simulink model "Neurofeedback_Fuzzy_full_fNIRS_pressure"  (R2022a)
settings: Solver=VariableStepAuto  StartTime=0.0  StopTime=200  RelTol=1e-6
libraries: fuzblock x1, simulink x1
settings Model: Creator=mariodelossantos  LastModifiedBy=mariodelossantos

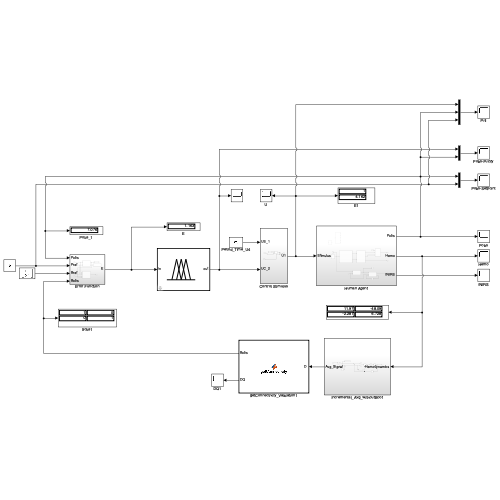
[thumbnail: Simulink's stored preview of the top-level diagram]
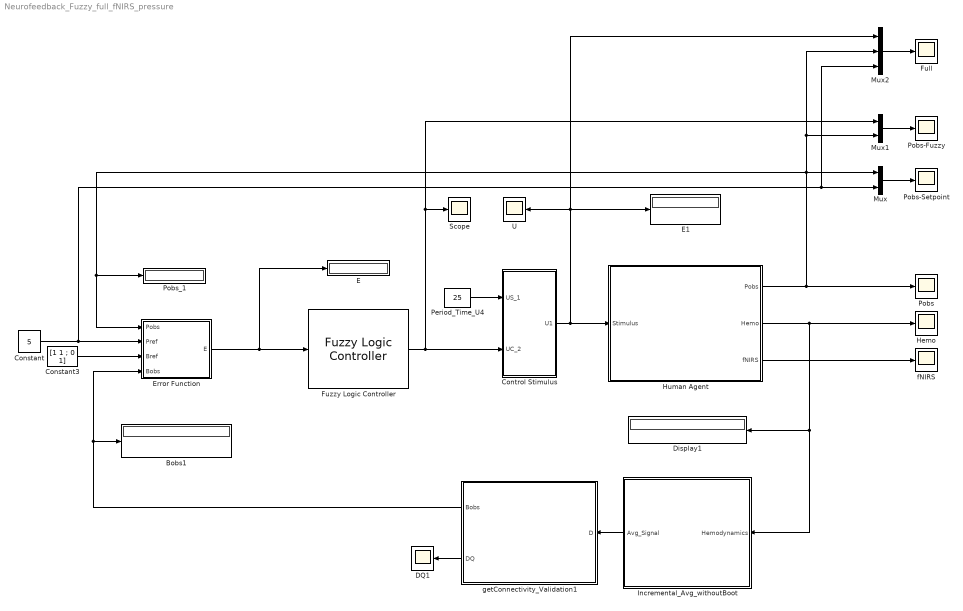
== system Neurofeedback_Fuzzy_full_fNIRS_pressure ==
  Bobs1 : Display
  Constant : Constant  Value=5
  Constant3 : Constant  Value="[1   1 ; 0  1]"
  Control Stimulus : Subsystem
  DQ1 : Scope
  Display1 : Display
  E : Display
  E1 : Display
  Error Function : Subsystem
  Full : Scope
  Fuzzy Logic Controller : fuzblock/Fuzzy Logic  Controller  FIS=cFNIRS  OutputSampleNumber=101  DataType=double  FuzzifiedInputs=off  RuleFiringStrengths=off  RuleOutputs=off  AggregatedOutputs=off  SimulateUsing=Interpreted execution  OutOfRangeInputValueMessage=warning  NoRuleFiredMessage=warning  EmptyOutputFuzzySetMessage=warning
  Hemo : Scope
  Human Agent : Subsystem
  Incremental_Avg_withoutBoot : Subsystem
  Mux : Mux  Inputs=2
  Mux1 : Mux  Inputs=2
  Mux2 : Mux  Inputs=3
  Period_Time_U4 : Constant  Value=25
  Pobs : Scope
  Pobs-Fuzzy : Scope
  Pobs-Setpoint : Scope
  Pobs_1 : Display
  Scope : Scope
  U : Scope
  fNIRS : Scope
  getConnectivity_Validation1 : MATLAB Function  TreatAsAtomicUnit=on  SystemSampleTime=0
  wires:
  Period_Time_U4/1 -> Control Stimulus/1(US_1)
  Error Function/1(E) -> Fuzzy Logic Controller/1, E/1
  Constant3/1 -> Error Function/3(Bref)
  getConnectivity_Validation1/1(Bobs) -> Error Function/4(Bobs), Bobs1/1
  Mux/1 -> Pobs-Setpoint/1
  Fuzzy Logic Controller/1 -> Mux1/1, Scope/1, Control Stimulus/2(UC_2)
  Constant/1 -> Mux/2, Mux2/3, Error Function/2(Pref)
  Human Agent/3(fNIRS) -> fNIRS/1
  Human Agent/2(Hemo) -> Hemo/1, Incremental_Avg_withoutBoot/1(Hemodynamics), Display1/1
  Incremental_Avg_withoutBoot/1(Avg_Signal) -> getConnectivity_Validation1/1("D ")
  Human Agent/1(Pobs) -> Mux2/2, Mux1/2, Error Function/1(Pobs), Pobs_1/1, Mux/1, Pobs/1
  getConnectivity_Validation1/2(DQ) -> DQ1/1
  Control Stimulus/1(U1) -> Mux2/1, U/1, E1/1, Human Agent/1(Stimulus)
  Mux1/1 -> Pobs-Fuzzy/1
  Mux2/1 -> Full/1

== system Neurofeedback_Fuzzy_full_fNIRS_pressure/Control Stimulus ==
  US_1 : Inport
  UC_2 : Inport  Port=2
  Duty_Cycle_U1 : Constant  Value=0.2  OutMin=[0]  OutMax=[0.8]
  Mux : Mux  Inputs=2
  Variable Pulse Generator2 : VariablePulseGenerator  RunAtFixedTimeIntervals=on  SampleTime=1/100
  U1 : Outport
  wires:
  Duty_Cycle_U1/1 -> Variable Pulse Generator2/1
  US_1/1 -> Variable Pulse Generator2/2
  Variable Pulse Generator2/1 -> Mux/1
  UC_2/1 -> Mux/2
  Mux/1 -> U1/1

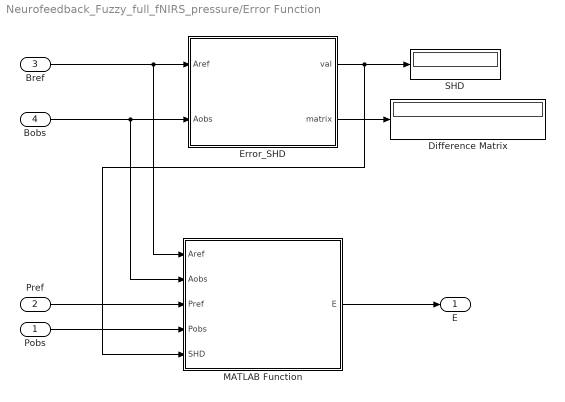
== system Neurofeedback_Fuzzy_full_fNIRS_pressure/Error Function ==
  Pobs : Inport
  Pref : Inport  Port=2
  Bref : Inport  Port=3
  Bobs : Inport  Port=4
  Difference Matrix : Display
  Error_SHD : MATLAB Function  TreatAsAtomicUnit=on
  MATLAB Function : MATLAB Function  TreatAsAtomicUnit=on
  SHD : Display
  E : Outport
  wires:
  Error_SHD/2(matrix) -> Difference Matrix/1
  Bref/1 -> MATLAB Function/1(Aref), Error_SHD/1(Aref)
  Error_SHD/1(val) -> SHD/1, MATLAB Function/5(SHD)
  MATLAB Function/1(E) -> E/1
  Bobs/1 -> MATLAB Function/2(Aobs), Error_SHD/2(Aobs)
  Pobs/1 -> MATLAB Function/4(Pobs)
  Pref/1 -> MATLAB Function/3(Pref)

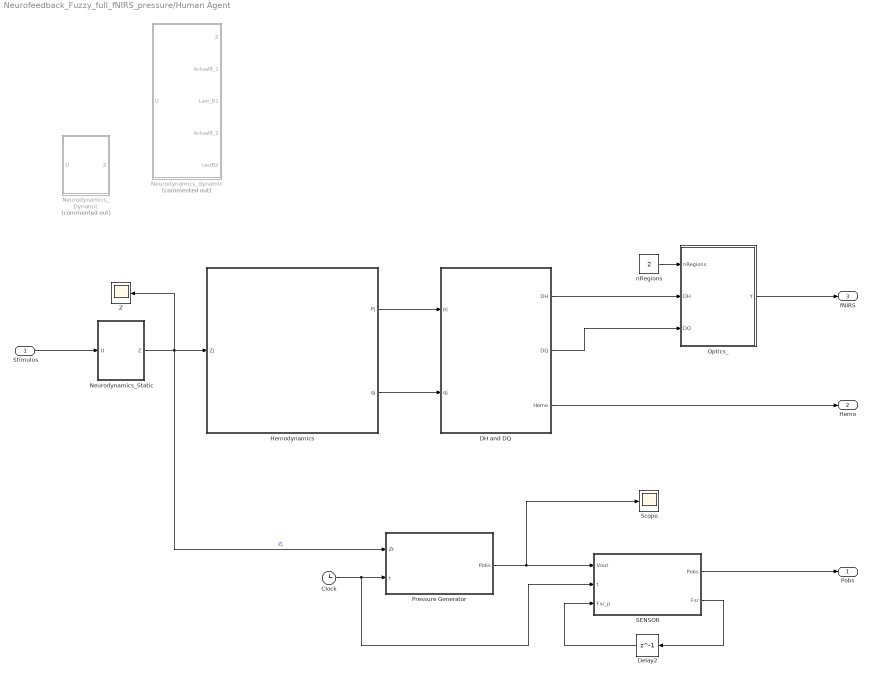
== system Neurofeedback_Fuzzy_full_fNIRS_pressure/Human Agent ==
  Stimulus : Inport
  Clock : Clock
  DH and DQ : Subsystem
  Delay2 : Delay  DelayLength=1  InitialCondition=0.0001
  Hemodynamics : Subsystem
  Neurodynamics_Dynamic : Subsystem  Commented=on
  Neurodynamics_Static : Subsystem
  Neurodynamics_dynamic : Subsystem  Commented=on
  Optics_ : MATLAB Function  TreatAsAtomicUnit=on
  Pressure Generator : MATLAB Function  TreatAsAtomicUnit=on
  SENSOR : MATLAB Function  TreatAsAtomicUnit=on
  Scope : Scope
  Z : Scope
  nRegions : Constant  Value=2
  Pobs : Outport
  Hemo : Outport  Port=2
  fNIRS : Outport  Port=3
  wires:
  Hemodynamics/1(Pj) -> DH and DQ/1(pj)
  Hemodynamics/2(qj) -> DH and DQ/2(qj)
  DH and DQ/1(DH) -> Optics_/2(DH)
  DH and DQ/2(DQ) -> Optics_/3(DQ)
  Pressure Generator/1(Pobs) -> Scope/1, SENSOR/1(Vout)
  Delay2/1 -> SENSOR/3(Fsr_p)
  SENSOR/2(Fsr) -> Delay2/1
  SENSOR/1(Pobs) -> Pobs/1
  Clock/1 -> Pressure Generator/2(t), SENSOR/2(t)
  Neurodynamics_Static/1(Z) -> Pressure Generator/1(Zt), Z/1, Hemodynamics/1(Zj)  "Zj"
  Stimulus/1 -> Neurodynamics_Static/1(U)
  nRegions/1 -> Optics_/1(nRegions)
  Optics_/1(Y) -> fNIRS/1
  DH and DQ/3(Hemo) -> Hemo/1

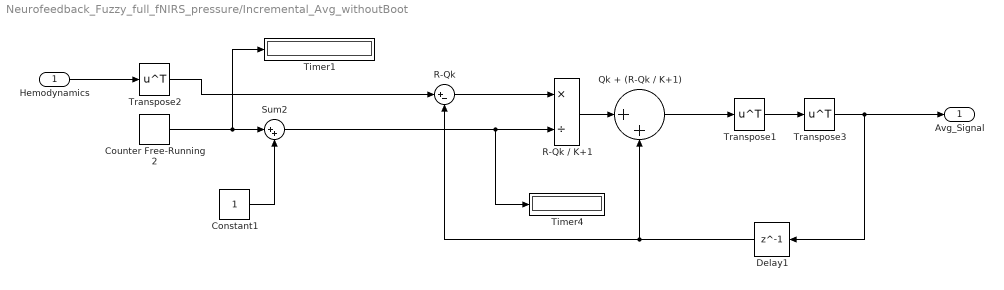
== system Neurofeedback_Fuzzy_full_fNIRS_pressure/Incremental_Avg_withoutBoot ==
  Hemodynamics : Inport
  Constant1 : Constant
  Counter Free-Running2 : simulink/Sources/Counter Free-Running  NumBits=32  tsamp=-1
  Delay1 : Delay  DelayLength=1  InitialCondition=[0 0 0 0]
  "Qk + (R-Qk / K+1) " : Sum  Inputs=|++
  R-Qk : Sum  Inputs=|+-
  R-Qk / K+1 : Product  Inputs=*/
  Sum2 : Sum  Inputs=|++
  Timer1 : Display
  Timer4 : Display
  Transpose1 : Math  Operator=transpose
  Transpose2 : Math  Operator=transpose
  Transpose3 : Math  Operator=transpose
  Avg_Signal : Outport
  wires:
  Constant1/1 -> Sum2/2
  Transpose2/1 -> R-Qk/1
  R-Qk / K+1/1 -> "Qk + (R-Qk / K+1) "/1
  "Qk + (R-Qk / K+1) "/1 -> Transpose1/1
  Hemodynamics/1 -> Transpose2/1
  Sum2/1 -> Timer4/1, R-Qk / K+1/2
  R-Qk/1 -> R-Qk / K+1/1
  Delay1/1 -> R-Qk/2, "Qk + (R-Qk / K+1) "/2
  Counter Free-Running2/1 -> Timer1/1, Sum2/1
  Transpose1/1 -> Transpose3/1
  Transpose3/1 -> Delay1/1, Avg_Signal/1

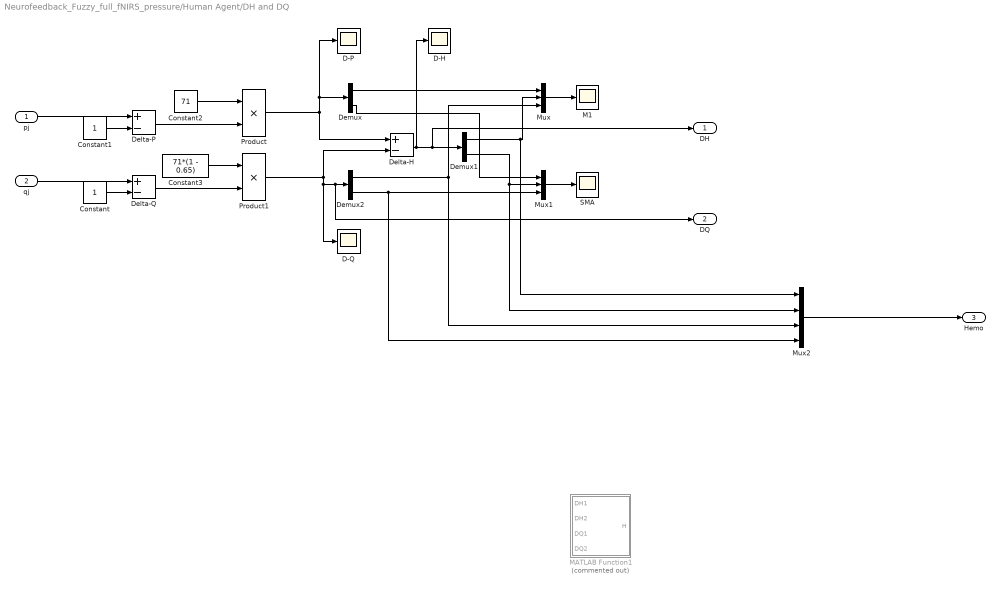
== system Neurofeedback_Fuzzy_full_fNIRS_pressure/Human Agent/DH and DQ ==
  pj : Inport
  qj : Inport  Port=2
  Constant : Constant
  Constant1 : Constant
  Constant2 : Constant  Value=71
  Constant3 : Constant  Value=71*(1 - 0.65)
  D-H : Scope
  D-P : Scope
  D-Q : Scope
  Delta-H : Sum  Inputs=+-
  Delta-P : Sum  Inputs=+-
  Delta-Q : Sum  Inputs=+-
  Demux : Demux  Outputs=2
  Demux1 : Demux  Outputs=2
  Demux2 : Demux  Outputs=2
  M1 : Scope
  MATLAB Function1 : MATLAB Function  Commented=on  TreatAsAtomicUnit=on
  Mux : Mux  Inputs=3
  Mux1 : Mux  Inputs=3
  Mux2 : Mux
  Product : Product
  Product1 : Product
  SMA : Scope
  DH : Outport
  DQ : Outport  Port=2
  Hemo : Outport  Port=3
  wires:
  Constant2/1 -> Product/1
  Delta-Q/1 -> Product1/2
  Constant3/1 -> Product1/1
  Demux2/2 -> Mux2/4, Mux1/3
  pj/1 -> Delta-P/1
  Mux1/1 -> SMA/1
  Demux/2 -> Mux1/1
  Mux/1 -> M1/1
  Constant/1 -> Delta-Q/2
  Delta-P/1 -> Product/2
  Product1/1 -> DQ/1, Demux2/1, D-Q/1, Delta-H/2
  qj/1 -> Delta-Q/1
  Demux/1 -> Mux/1
  Delta-H/1 -> DH/1, Demux1/1, D-H/1
  Demux1/1 -> Mux2/1, Mux/2
  Demux1/2 -> Mux2/2, Mux1/2
  Product/1 -> Demux/1, D-P/1, Delta-H/1
  Demux2/1 -> Mux2/3, Mux/3
  Constant1/1 -> Delta-P/2
  Mux2/1 -> Hemo/1

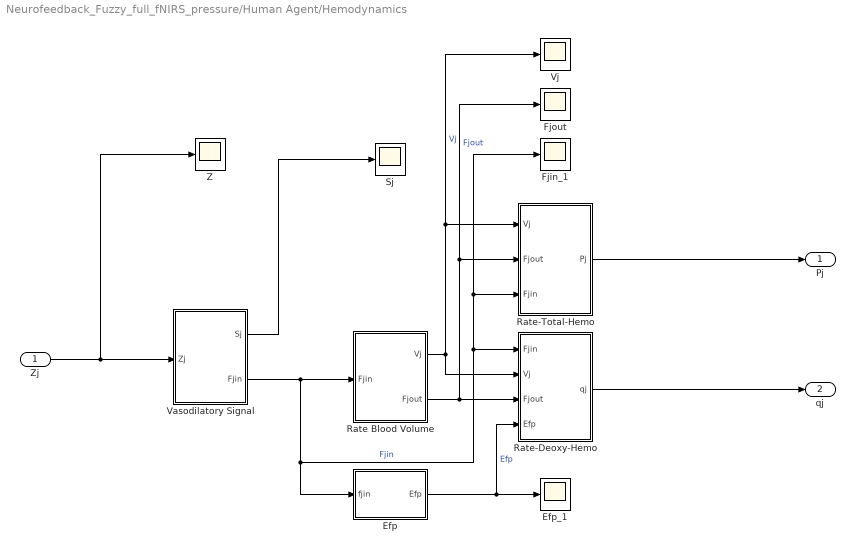
== system Neurofeedback_Fuzzy_full_fNIRS_pressure/Human Agent/Hemodynamics ==
  Zj : Inport
  Efp : MATLAB Function  TreatAsAtomicUnit=on
  Efp_1 : Scope
  Fjin_1 : Scope
  Fjout : Scope
  Rate Blood Volume : Subsystem
  Rate-Deoxy-Hemo : Subsystem
  Rate-Total-Hemo : Subsystem
  Sj : Scope
  Vasodilatory Signal : Subsystem
  Vj : Scope
  Z : Scope
  Pj : Outport
  qj : Outport  Port=2
  wires:
  Rate-Deoxy-Hemo/1(qj) -> qj/1
  Zj/1 -> Vasodilatory Signal/1(Zj), Z/1
  Vasodilatory Signal/1(Sj) -> Sj/1
  Rate Blood Volume/2(Fjout) -> Fjout/1, Rate-Total-Hemo/2(Fjout), Rate-Deoxy-Hemo/3(Fjout)  "Fjout"
  Rate Blood Volume/1(Vj) -> Vj/1, Rate-Total-Hemo/1(Vj), Rate-Deoxy-Hemo/2(Vj)  "Vj"
  Rate-Total-Hemo/1(Pj) -> Pj/1
  Efp/1(Efp) -> Rate-Deoxy-Hemo/4(Efp), Efp_1/1  "Efp"
  Vasodilatory Signal/2(Fjin) -> Efp/1(fjin), Fjin_1/1, Rate-Total-Hemo/3(Fjin), Rate-Deoxy-Hemo/1(Fjin), Rate Blood Volume/1(Fjin)  "Fjin"

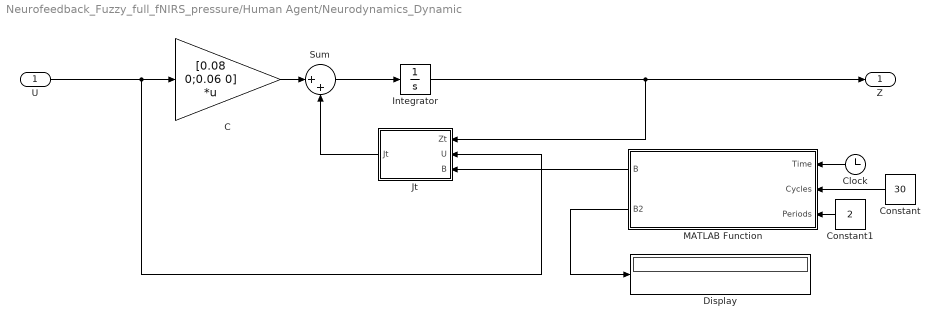
== system Neurofeedback_Fuzzy_full_fNIRS_pressure/Human Agent/Neurodynamics_Dynamic ==
  U : Inport
  C : Gain  Gain=[0.08 0;0.06 0]  Multiplication=Matrix(K*u) (u vector)
  Clock : Clock
  Constant : Constant  Value=30
  Constant1 : Constant  Value=2
  Display : Display
  Integrator : Integrator
  Jt : MATLAB Function  TreatAsAtomicUnit=on
  MATLAB Function : MATLAB Function  TreatAsAtomicUnit=on
  Sum : Sum  Inputs=|++
  Z : Outport
  wires:
  C/1 -> Sum/1
  Jt/1(Jt) -> Sum/2
  Sum/1 -> Integrator/1
  Constant1/1 -> MATLAB Function/3(Periods)
  Clock/1 -> MATLAB Function/1(Time)
  Constant/1 -> MATLAB Function/2(Cycles)
  MATLAB Function/2(B2) -> Display/1
  MATLAB Function/1(B) -> Jt/3(B)
  U/1 -> C/1, Jt/2(U)
  Integrator/1 -> Z/1, Jt/1(Zt)

== system Neurofeedback_Fuzzy_full_fNIRS_pressure/Human Agent/Neurodynamics_Static ==
  U : Inport
  C : Gain  Gain=[0.08 0;0.06 0]  Multiplication=Matrix(K*u)
  Integrator : Integrator
  Jt : MATLAB Function  TreatAsAtomicUnit=on
  Sum : Sum  Inputs=|++
  Z : Outport
  wires:
  Integrator/1 -> Z/1, Jt/1(Zt)
  C/1 -> Sum/1
  Jt/1(Jt) -> Sum/2
  Sum/1 -> Integrator/1
  U/1 -> C/1, Jt/2(U)

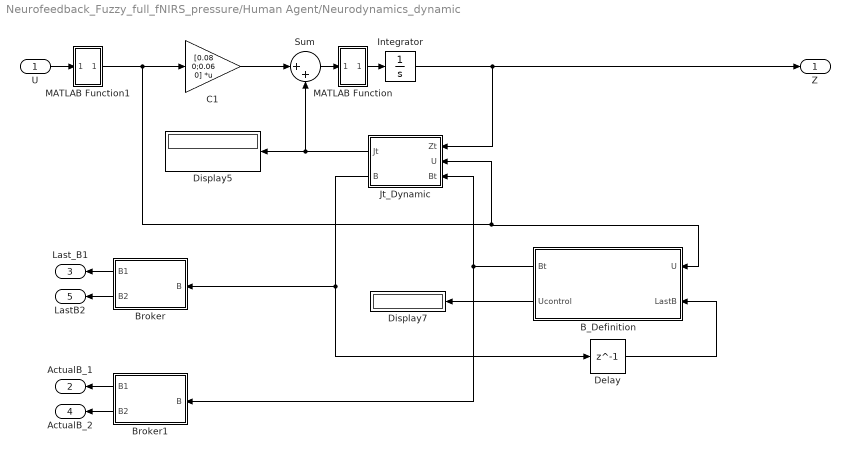
== system Neurofeedback_Fuzzy_full_fNIRS_pressure/Human Agent/Neurodynamics_dynamic ==
  U : Inport
  B_Definition : MATLAB Function  TreatAsAtomicUnit=on
  Broker : MATLAB Function  TreatAsAtomicUnit=on
  Broker1 : MATLAB Function  TreatAsAtomicUnit=on
  C1 : Gain  Gain=[0.08 0;0.06 0]  Multiplication=Matrix(K*u) (u vector)
  Delay : Delay  DelayLength=1  InitialCondition=0
  Display5 : Display
  Display7 : Display
  Integrator : Integrator
  Jt_Dynamic : MATLAB Function  TreatAsAtomicUnit=on
  MATLAB Function : MATLAB Function  TreatAsAtomicUnit=on
  MATLAB Function1 : MATLAB Function  TreatAsAtomicUnit=on
  Sum : Sum  Inputs=|++
  Z : Outport
  ActualB_1 : Outport  Port=2
  Last_B1 : Outport  Port=3
  ActualB_2 : Outport  Port=4
  LastB2 : Outport  Port=5
  wires:
  Integrator/1 -> Z/1, Jt_Dynamic/1(Zt)
  C1/1 -> Sum/1
  U/1 -> MATLAB Function1/1(Z)
  Sum/1 -> MATLAB Function/1(Z)
  MATLAB Function1/1(Zn) -> C1/1, B_Definition/1(U), Jt_Dynamic/2(U)
  MATLAB Function/1(Zn) -> Integrator/1
  Jt_Dynamic/1(Jt) -> Display5/1, Sum/2
  Delay/1 -> B_Definition/2(LastB)
  Jt_Dynamic/2(B) -> Broker/1(B), Delay/1
  B_Definition/1(Bt) -> Jt_Dynamic/3(Bt), Broker1/1(B)
  B_Definition/2(Ucontrol) -> Display7/1
  Broker1/1(B1) -> ActualB_1/1
  Broker1/2(B2) -> ActualB_2/1
  Broker/2(B2) -> LastB2/1
  Broker/1(B1) -> Last_B1/1

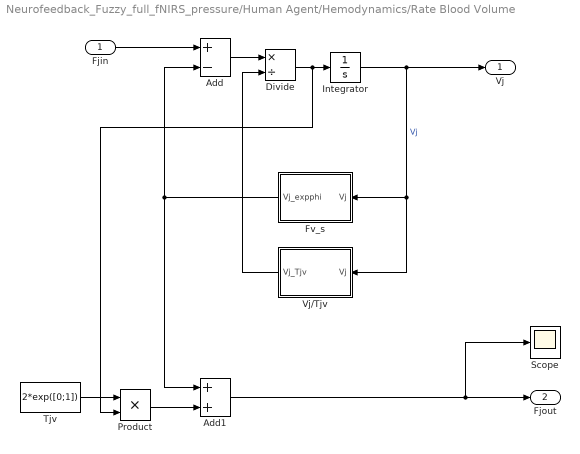
== system Neurofeedback_Fuzzy_full_fNIRS_pressure/Human Agent/Hemodynamics/Rate Blood Volume ==
  Fjin : Inport
  Add : Sum  Inputs=+-
  Add1 : Sum
  Divide : Product  Inputs=*/
  Fv_s : MATLAB Function  TreatAsAtomicUnit=on
  Integrator : Integrator  InitialCondition=exp([0;0])
  Product : Product
  Scope : Scope
  Tjv : Constant  Value=2*exp([0;1])
  Vj/Tjv : MATLAB Function  TreatAsAtomicUnit=on
  Vj : Outport
  Fjout : Outport  Port=2
  wires:
  Fjin/1 -> Add/1
  Integrator/1 -> Vj/1, Vj/Tjv/1(Vj), Fv_s/1(Vj)  "Vj"
  Divide/1 -> Product/2, Integrator/1
  Fv_s/1(Vj_expphi) -> Add/2, Add1/1
  Add/1 -> Divide/1
  Vj/Tjv/1(Vj_Tjv) -> Divide/2
  Product/1 -> Add1/2
  Tjv/1 -> Product/1
  Add1/1 -> Scope/1, Fjout/1

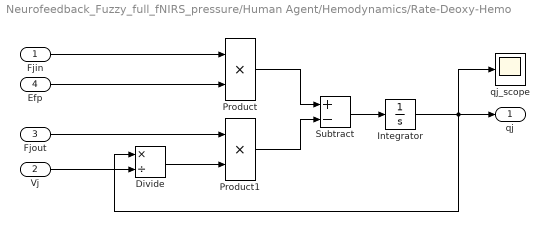
== system Neurofeedback_Fuzzy_full_fNIRS_pressure/Human Agent/Hemodynamics/Rate-Deoxy-Hemo ==
  Fjin : Inport
  Vj : Inport  Port=2
  Fjout : Inport  Port=3
  Efp : Inport  Port=4
  Divide : Product  Inputs=*/
  Integrator : Integrator  InitialCondition=exp([0;0])
  Product : Product
  Product1 : Product
  Subtract : Sum  Inputs=+-
  qj_scope : Scope
  qj : Outport
  wires:
  Efp/1 -> Product/2
  Divide/1 -> Product1/2
  Subtract/1 -> Integrator/1
  Integrator/1 -> qj/1, Divide/1, qj_scope/1
  Vj/1 -> Divide/2
  Product1/1 -> Subtract/2
  Fjin/1 -> Product/1
  Fjout/1 -> Product1/1
  Product/1 -> Subtract/1

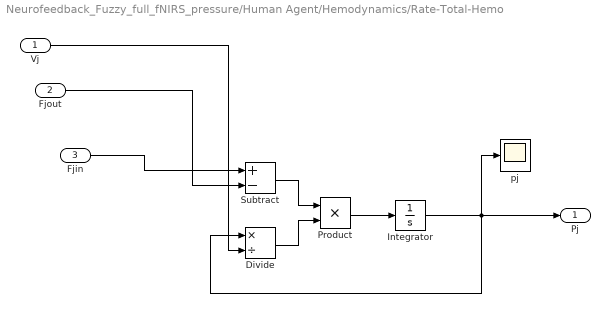
== system Neurofeedback_Fuzzy_full_fNIRS_pressure/Human Agent/Hemodynamics/Rate-Total-Hemo ==
  Vj : Inport
  Fjout : Inport  Port=2
  Fjin : Inport  Port=3
  Divide : Product  Inputs=*/
  Integrator : Integrator  InitialCondition=exp([0;0])
  Product : Product
  Subtract : Sum  Inputs=+-
  pj : Scope
  Pj : Outport
  wires:
  Fjout/1 -> Subtract/2
  Product/1 -> Integrator/1
  Vj/1 -> Divide/2
  Subtract/1 -> Product/1
  Fjin/1 -> Subtract/1
  Divide/1 -> Product/2
  Integrator/1 -> Pj/1, pj/1, Divide/1

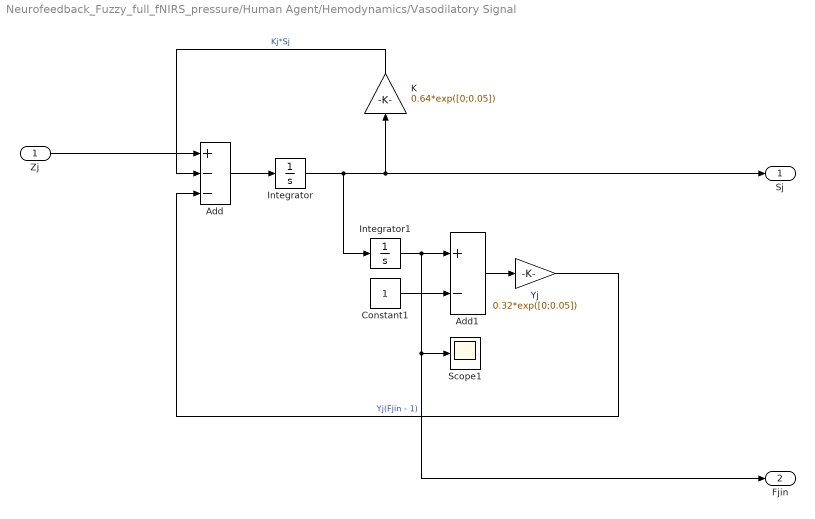
== system Neurofeedback_Fuzzy_full_fNIRS_pressure/Human Agent/Hemodynamics/Vasodilatory Signal ==
  Zj : Inport
  Add : Sum  Inputs=+--
  Add1 : Sum  Inputs=+-
  Constant1 : Constant
  Integrator : Integrator
  Integrator1 : Integrator  InitialCondition=exp([0;0])
  K : Gain  Gain=0.64*exp([0;0.05])
  Scope1 : Scope
  Yj : Gain  Gain=0.32*exp([0;0.05])
  Sj : Outport
  Fjin : Outport  Port=2
  wires:
  Add1/1 -> Yj/1
  K/1 -> Add/2  "Kj*Sj"
  Constant1/1 -> Add1/2
  Zj/1 -> Add/1
  Integrator1/1 -> Fjin/1, Scope1/1, Add1/1
  Integrator/1 -> Sj/1, K/1, Integrator1/1
  Add/1 -> Integrator/1
  Yj/1 -> Add/3  "Yj(Fjin - 1)"

== matlab function Neurofeedback_Fuzzy_full_fNIRS_pressure/Human Agent/Neurodynamics_dynamic/Broker ==
  data: B input; B1 output; B2 output
function [B1, B2] = fcn(B)
B1 = B(:,:,1);
B2 = B(:,:,2);

== matlab function Neurofeedback_Fuzzy_full_fNIRS_pressure/Human Agent/Neurodynamics_dynamic/Broker1 ==
  data: B input; B1 output; B2 output
function [B1, B2] = fcn(B)
B1 = B(:,:,1);
B2 = B(:,:,2);

== matlab function Neurofeedback_Fuzzy_full_fNIRS_pressure/Human Agent/Pressure Generator ==
  data: Zt input; Pobs output; t input
function Pobs = fcn(Zt, t)
    R=1000; %Resistor [Ohms];
    C= 1.5; %Capacitor [Faradays];
    V= Zt(1); %Voltage or system reference;
    Vc = V * (exp(-t/(R*C))); % Voltage at the capacitor  
    
Pobs = Vc;

== matlab function Neurofeedback_Fuzzy_full_fNIRS_pressure/Human Agent/Neurodynamics_dynamic/Jt_Dynamic ==
  data: Zt input; U input; Jt output; Bt input; B output
function [Jt, B] = fcn(Zt, U, Bt)

   A = [-0.16 -0.49;-0.02 -0.33];
   nRegions  = size(A,1);

   B = zeros(2,2,2);
   a = 0;
   B1 = [0 0; 0 0]; %There must be a B per stimulus
   B2 = [-0.02 -0.77; 0.33 -1.31];

   if Bt(:,:,2) ~= B(:,:,2)
       B(:,:,:) = Bt(:,:,:);
   else
          B(:,:,1) = B1;
          B(:,:,2) = B2;
   end
   M = size(U,1); %nStimuli
   assert(M == size(B,3),...
        'Unexpected number of induced connectivity parameters B.');

    simulationLength = size(U,2);
    for t = 1:simulationLength
       T = zeros(nRegions); %nRegions x nRegions
                   for uu = 1:M % Sum (Uj * Bj)
                       tmp = U(uu,t) * B(:,:,uu);
                       T = -0.5 * exp(T + tmp);  
                   end
            SI = diag(A);
    end
        A =  A - diag(exp(SI) + (SI));
Jt = (A*Zt) + (T*Zt);

== matlab function Neurofeedback_Fuzzy_full_fNIRS_pressure/Human Agent/Hemodynamics/Efp ==
  data: fjin input; Efp output
function Efp= fcn(fjin)

Efp = (1 - (1 - 0.32).^ (1 ./ fjin))/0.32;

== matlab function Neurofeedback_Fuzzy_full_fNIRS_pressure/Human Agent/Neurodynamics_dynamic/MATLAB Function ==
  data: Z input; Zn output
function Zn = fcn(Z)

Zn = Z(:,1);

== matlab function Neurofeedback_Fuzzy_full_fNIRS_pressure/Human Agent/Neurodynamics_dynamic/MATLAB Function1 ==
  data: Z input; Zn output
function Zn = fcn(Z)

Zn = Z(:,1);

== matlab function Neurofeedback_Fuzzy_full_fNIRS_pressure/Human Agent/SENSOR ==
  data: Vout input; Pobs output; t input; Fsr_p input; Fsr output
function [Pobs,Fsr] = PressureGenerator_sensor(Vout, t,Fsr_p)

    Vcc = 50; %Considering 5V as a real sensor, the value is on mV
    Rf = 100; %Fixed resistor 10k ohms
    kgf = 0.1019716213; % 1N = 0.1019716213 kgf
    Fsr = 0;
    Fsrforce = 0;
    Fsr = (Vcc - Vout * Rf) / Vout;
    FsConductance = 1000000; %Sensor conductance in uOhms
    FsConductance = FsConductance / Fsr;
    if FsConductance <= 1000
        Fsrforce = FsConductance / 80; %Force on Newtons
    else
        Fsrforce = FsConductance - 1000;
        Fsrforce = Fsrforce / 30;
    end
    
Pobs = Fsrforce * kgf;

end

== matlab function Neurofeedback_Fuzzy_full_fNIRS_pressure/Human Agent/DH and DQ/MATLAB Function1 ==
  data: DH1 input; H output; DH2 input; DQ1 input; DQ2 input
function H = hemo(DH1, DH2, DQ1, DQ2)
H = zeros(1,4);

H(1,1) = DQ1;
H(1,2) = DQ2;
H(1,3) = DH1;
H(1,4) = DH2;

== matlab function Neurofeedback_Fuzzy_full_fNIRS_pressure/Human Agent/Hemodynamics/Rate Blood Volume/Fv_s ==
  data: Vj input; Vj_expphi output
function Vj_expphi = fcn(Vj)
phi = 0.32;
Vj_expphi = Vj.^(1/phi);

== matlab function Neurofeedback_Fuzzy_full_fNIRS_pressure/Error Function/Error_SHD ==
  data: Aref input; val output; Aobs input; matrix output
function [val,matrix]=SHD(Aref,Aobs)

val = sum(sum(xor(Aref,Aobs)));
matrix = xor(Aref,Aobs);

== matlab function Neurofeedback_Fuzzy_full_fNIRS_pressure/Human Agent/Hemodynamics/Rate Blood Volume/Vj//Tjv ==
  data: Vj input; Vj_Tjv output
function Vj_Tjv = fcn(Vj)
    Tjv = 2*exp([0;1]);
    Tj = 2*exp([0;0.05]);
Vj_Tjv =(Tj.*Tjv.*Vj);

== matlab function Neurofeedback_Fuzzy_full_fNIRS_pressure/Error Function/MATLAB Function ==
  data: Aref input; E output; Aobs input; Pref input; Pobs input; SHD input
function E  = ErrorFunction(Aref, Aobs, Pref, Pobs, SHD)
    w1 = 0.5; %Use whatever values you like most. Threshold 

    w2 = 1 - w1;

    assert(all(size(Aref) == size(Aobs)));

    assert(size(Aref,1) == size(Aref,2));

    nChannels = size(Aref,1);

    AfullyConnected = ones(nChannels);

    AfullyDisconnected = zeros(nChannels);

    maxDiffSHD = sum(sum(xor(AfullyConnected,AfullyDisconnected))); %SHD

    errA = SHD/maxDiffSHD; %Normalize error in the connectivity

    errP = abs(Pref-Pobs);

    
E = w1 * errA + w2 * errP;

== matlab function Neurofeedback_Fuzzy_full_fNIRS_pressure/getConnectivity_Validation1 ==
  data: D input; Bobs output; DQ output
function [Bobs,DQ]  = getConnectivity(D)

    DQ = zeros(1, 2);
    DQ(1,1)=D(1,1);
    DQ(1,2)=D(1,2);


    DH = zeros(1,2);
    DH(1,1)=D(1,3);
    DH(1,2)=D(1,4);

    rThresh= 0.6; % [0..1] A threshold on the correlation.

    [nSamples,nChannels, nHb]=size(DQ);

    C = nan(nChannels, nChannels, nHb); %Matrix of channel pairwise correlations;

    %This part of the algorithm is HIGHLY inefficient but it does the job for now
    %but might not be sufficiently fast for "real time" neurofeedback

    for iHb = 1:nHb
        for iCh=1:nChannels
            for jCh=iCh:nChannels

                if iCh == jCh

                 C(iCh,jCh,iHb) = 1;

                else

                 C(iCh,jCh,iHb) = xcorr2(DQ(:,iCh,iHb),DQ(:,jCh,iHb));

                end
            end

        end

    end

    %Threshold/Binarize C


    tmp = C > rThresh;

    %Finally "merge" accross Hb species

    Bobs = all(tmp,3); %Apply the AND function across Hb species.

== matlab function Neurofeedback_Fuzzy_full_fNIRS_pressure/Human Agent/Neurodynamics_Static/Jt ==
  data: Zt input; U input; Jt output
function Jt = fcn(Zt, U)
   A = [-0.16 -0.49;-0.02 -0.33];
   nRegions  = size(A,1);
   M = size(U,1); %nStimuli
   simulationLength = size(U,2);
   B = zeros(2,2,2);
   B1 = [0 0; 0 0]; %There must be a B per stimulus
   B2 = [-0.02 -0.77; 0.33 -1.31];
   %B2 = [1 1; 1 1];
   B(:,:,1) = B1;
   B(:,:,2) = B2;
      assert(M == size(B,3),...
       'Unexpected number of induced connectivity parameters B.');
   T = zeros(nRegions); %nRegions x nRegions
    for t = 1:simulationLength
           for uu = 1:M % Sum (Uj * Bj)
               tmp = U(uu,t)*B(:,:,uu);
               T = -0.5*exp(T + tmp);  
           end
    end
    SI = diag(A);
    A =  A - diag(exp(SI) + (SI));
Jt = (A*Zt) + (T*Zt);

== matlab function Neurofeedback_Fuzzy_full_fNIRS_pressure/Human Agent/Neurodynamics_Dynamic/Jt ==
  data: Zt input; U input; Jt output; B input
function Jt = fcn(Zt, U,B)
   A = [-0.16 -0.49;-0.02 -0.33];
   nRegions  = size(A,1);
   M = size(U,1); %nStimuli
   simulationLength = size(U,2);
%    B = zeros(2,2,2);
%    B1 = [0 0; 0 0]; %There must be a B per stimulus
%    %B2_3
%    B2 = [-0.67 -0.91 ;-0.3 -1.21];
%    %B2_2
%    %B2 = [-0.08 -1.08; 1.2054 -0.0076];
%    %B2_1
%    %B2 = [-0.02 -0.07; 0.33 -1.31];
%    B(:,:,1) = B1;
%    B(:,:,2) = B2;
      assert(M == size(B,3),...
       'Unexpected number of induced connectivity parameters B.');
   T = zeros(nRegions); %nRegions x nRegions
    for t = 1:simulationLength
           for uu = 1:M % Sum (Uj * Bj)
               tmp = U(uu,t)*B(:,:,uu);
               T = -0.5*exp(T + tmp);  
           end
    end
    SI = diag(A);
    A =  A - diag(exp(SI) + (SI));
Jt = (A*Zt) + (T*Zt);

== matlab function Neurofeedback_Fuzzy_full_fNIRS_pressure/Human Agent/Neurodynamics_Dynamic/MATLAB Function ==
  settings: updateMethod=DISCRETE
  data: Time input; B output; Cycles input; Periods input; B2 output
function [B, B2] = ControlledDynamic_B(Time, Cycles, Periods)

   B = zeros(2,2,2);
   %B1 = [0 0; 0 0]; %There must be a B per stimulus
   %B2_3
   %B2 = [-0.67 -0.91 ;-0.3 -1.21];
   %B2_2
   %B2 = [-0.08 -1.08; 1.2054 -0.0076];
   %B2_1
   %B2 = [-0.02 -0.07; 0.33 -1.31];
   PCycles = zeros(6,1);
   for i = 1:Periods
       PCycles(i) = i * Cycles;   
   end
   %random_selector = randi([1,3]);

   if(Time >= 0 && Time <= PCycles(2))
%       random_selector = randi([1,3]);
%       if(random_selector == 1)
          B1 = [0 0; 0 0];
          B2 = [-0.02 -0.07; 0.33 -1.31]; 
%       elseif(random_selector == 2)
%           B1 = [0 0; 0 0];
%           B2 = [-0.08 -1.08; 1.2054 -0.0076];
%       else
%           B1 = [0 0; 0 0];
%           B2 = [-0.67 -0.91; 0.3 -1.21];
      B(:,:,1) = B1;
      B(:,:,2) = B2;
   elseif(Time >= PCycles(2)+1 && Time <= PCycles(4))
       B1 = [0 0;0 0];
       B2 = [-0.08 -1.08; 1.2054 -0.0076];
       B(:,:,1) = B1;
       B(:,:,2) = B2;
   else
       B1 = [0 0; 0 0];
       B2 = [-0.67 -0.91; -0.3 -1.21];
       B(:,:,1) = B1;
       B(:,:,2) = B2;
   end

== matlab function Neurofeedback_Fuzzy_full_fNIRS_pressure/Human Agent/Optics_ ==
  data: nRegions input; DH input; DQ input; Y output
function Y = Optical_Changes(nRegions,DH, DQ)
%% Version V1
% Authors - Mario De Los Santos, Felipe Orihuela-Espina, Javier Herrara-Vega
% Date - March, 2022
% Email - madlsh3517@gmail.com
% Based on: 2015 Stak DCM for fNIRS.
%
%% Input Parameters
% DQ - HbR - Rate of deoxy-hemoglobin
% DH - HbT - Total Hemoglobin
%
%% Output Parameters
% y- optical density changes 
%
%% 

%Using simulink is not possible to have a dynamic matrix that we can
%iterate based on the nRegions variable, but you could easly replace the
%number of regions in the variable "Regions" according your needs
Regions = 2;
Y = zeros(Regions,Regions);
tempDHQ = zeros(nRegions, 2);


% We are using as L1 = 780nm and as L2 = 850nm (same as STak for the
% second one)
%Based on: Giannoni, L., Lange, F., & Tachtsidis, I. (2020). Investigation of the quantification 
% of hemoglobin and cytochrome-c-oxidase in the exposed cortex with near-infrared hyperspectral imaging: 
% a simulation study. Journal of biomedical optics, 25(4), 046001.

F_P =[(0.0007358251*7.5) (0.001104715*6.5) ; (0.001159306*7.5) (0.0007858993*6.5)]; 

%Itereation between regions, nRegions is given as constant by the user.
for i = 1:nRegions
    tempDHQ(:,i) = DQ(i);
    tempDHQ(:,i) = DH(i);
    Y(:,:) = F_P * tempDHQ;
end

== matlab function Neurofeedback_Fuzzy_full_fNIRS_pressure/Human Agent/Neurodynamics_dynamic/B_Definition ==
  settings: updateMethod=DISCRETE
  data: U input; Bt output; LastB input; Ucontrol output
function [Bt, Ucontrol] = B_Definition(U, LastB)
   Bt = zeros(2, 2, 2);
   %Control extraction and weight
   Ucontrol = U(2) * (0.2 + rand(1) * (1-0.2));
   Threshold = 0.2;
    if(Ucontrol < Threshold) %Random Ucontrol to test
        min = -1; 
        max = 1.5;
        n = 2;
        r1 = min + rand(n)*(max-min);
        r2 = min + rand(n)*(max-min);
        %Bt(:,:,1) = r1(:,:);
        Bt(:,:,2) = r2(:,:);
    else
       Bt = LastB;
    end
